simulink model "LQR"  (R2025b)
settings: Solver=VariableStepAuto  StartTime=0.0  StopTime=10  RelTol=1e-5
InitFcn:
  | clear; clc; close all;
  | 
  | % --- 1. System Parameters ---
  | m = 0.2;
  | M = 1;
  | g = 9.81;
  | bc = 0.1;
  | bp = 0.05;
  | l0 = 0.5;
  | theta0 = 0;
  | x0 = -0.5; % or -5
  | 
  | % --- 2. State-Space Matrices ---
  | A = [0, 1, 0, 0;
  |      0, -bc / M, (m * g) / M, bp / (M * l0);
  |      0, 0, 0, 1;
  |      0, bc / (M * l0), -g * (M + m) / (M * l0), -bp * (M + m) / (M * m * l0 ^ 2)];
  | 
  | % Only the 1st column of B is used (Input: Force F)
  | B_LQR = [0; 1 / M; 0; -1 / (M * l0)];
  | 
  | % --- 3. LQR Design ---
  | Q = diag([1000, 10, 500, 10]);
  | R = 1;
  | 
  | % Calculate LQR Gain 'K' silently
  | K = lqr(A, B_LQR, Q, R); % 31.6228   14.0488  -17.7264    0.3611
model workspace (MAT data in the model file):
  Sig = Simulink.Signal
  Sig.Dimensions = -1
  Sig.DimensionsMode = 'auto'
  Sig.Complexity = 'auto'
  Sig.SampleTime = -1
  Sig.SamplingMode = 'auto'
  Sig.DataType = 'auto'
undefined symbols (not defined in the file or in its folder): L, X, Y, Z
libraries: sm_lib x13, nesl_utility x7
settings Model: Creator=JNemune  LastModifiedBy=JNemune

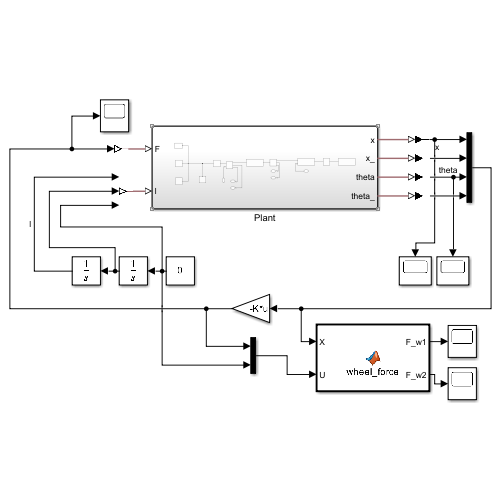
[thumbnail: Simulink's stored preview of the top-level diagram]
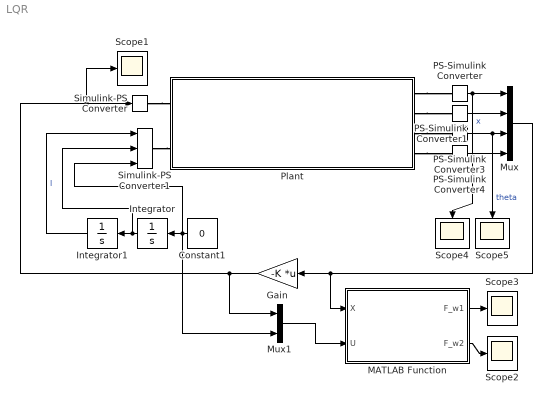
== system LQR ==
  Constant1 : Constant  Value=0
  Gain : Gain  Gain=-K  Multiplication=Matrix(K*u)
  Integrator : Integrator
  Integrator1 : Integrator  InitialCondition=l0
  MATLAB Function : MATLAB Function  TreatAsAtomicUnit=on
  Mux : Mux
  Mux1 : Mux  Inputs=2
  PS-Simulink Converter{,1,3..4} (4 alike) : nesl_utility/PS-Simulink Converter  PhysicalDomain=network_engine_domain  SubClassName=ps_output  LeftPortType=input  RightPortType=output  PseudoPeriodic=off  Frequencies=[]  VectorFormat=inherit  Unit=inherit  AffineConversion=off
  Plant : Subsystem
  Scope{1..5} (5 alike) : Scope
      Scope1 settings: Title=Plant Input (F, l_ddot)  ActiveDisplayYMinimum=-3.88186183734339  ActiveDisplayYMaximum=17.999527205084721
      Scope2 settings: Title=Plant Input (F, l_ddot)  ActiveDisplayYMinimum=5.7232322835325906  ActiveDisplayYMaximum=6.2250486767824951  DataLoggingVariableName=ScopeData2
      Scope3 settings: Title=Plant Input (F, l_ddot)  ActiveDisplayYMinimum=5.6634140711184715  ActiveDisplayYMaximum=6.09883492734478  DataLoggingVariableName=ScopeData3
      Scope4 settings: Title=Plant Input (F, l_ddot)  ActiveDisplayYMinimum=-0.56814105763095268  ActiveDisplayYMaximum=0.11326951867857375
      Scope5 settings: Title=Plant Input (F, l_ddot)  ActiveDisplayYMinimum=-0.29673612139259414  ActiveDisplayYMaximum=0.21369870792859819  DataLoggingVariableName=ScopeData4
  Simulink-PS Converter : nesl_utility/Simulink-PS Converter  PhysicalDomain=network_engine_domain  SubClassName=ps_input  LeftPortType=input  RightPortType=output  PseudoPeriodic=off  Frequencies=[]  NoiseDistribution=none  NoiseParameters=[]  Unit=1  AffineConversion=off  FilteringAndDerivatives=provide  SimscapeFilterOrder=1  InputFilterTimeConstant=0.001  UdotUserProvided=0
  Simulink-PS Converter1 : nesl_utility/Simulink-PS Converter  PhysicalDomain=network_engine_domain  SubClassName=ps_input  LeftPortType=input  RightPortType=output  PseudoPeriodic=off  Frequencies=[]  NoiseDistribution=none  NoiseParameters=[]  Unit=1  AffineConversion=off  FilteringAndDerivatives=provide  SimscapeFilterOrder=1  InputFilterTimeConstant=0.001  UdotUserProvided=2
  wires:
  Integrator/1 -> Simulink-PS Converter1/2, Integrator1/1
  Integrator1/1 -> Simulink-PS Converter1/1  "l"
  Constant1/1 -> Mux1/2, Simulink-PS Converter1/3, Integrator/1
  Gain/1 -> Mux1/1, Simulink-PS Converter/1, Scope1/1
  Mux/1 -> MATLAB Function/1(X), Gain/1
  PS-Simulink Converter1/1 -> Mux/2
  PS-Simulink Converter3/1 -> Scope5/1, Mux/3  "theta"
  PS-Simulink Converter4/1 -> Mux/4
  PS-Simulink Converter/1 -> Scope4/1, Mux/1  "x"
  Mux1/1 -> MATLAB Function/2(U)
  MATLAB Function/1(F_w1) -> Scope3/1
  MATLAB Function/2(F_w2) -> Scope2/1
  connections:
  Plant/RConn2 -- PS-Simulink Converter1/LConn1
  Simulink-PS Converter1/RConn1 -- Plant/LConn2
  Simulink-PS Converter/RConn1 -- Plant/LConn1
  Plant/RConn3 -- PS-Simulink Converter3/LConn1
  Plant/RConn1 -- PS-Simulink Converter/LConn1
  Plant/RConn4 -- PS-Simulink Converter4/LConn1

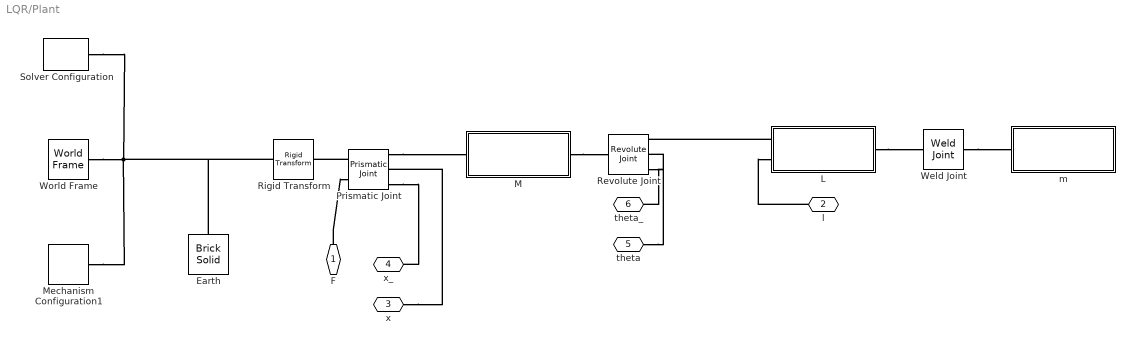
== system LQR/Plant ==
  Earth : sm_lib/Body Elements/Brick Solid  BrickDimensions=[1000 1 1]  BrickDimensionsUnits=mm  ExportEntireGeometry=off  InertiaType=CalculateFromGeometry  BasedOnType=Density  Density=1000  DensityUnits=kg/m^3  Mass=1  MassUnits=kg  CenterOfMass=[0 0 0]  CenterOfMassUnits=m  MomentsOfInertia=[1 1 1]  MomentsOfInertiaUnits=kg*m^2  ProductsOfInertia=[0 0 0]  ProductsOfInertiaUnits=kg*m^2  GraphicType=FromGeometry  MarkerShape=Sphere  MarkerSize=10  GraphicVisPropType=SimpleVisualProperties  GraphicDiffuseColor=[0.5 0.5 0.5]  GraphicOpacity=1.0  GraphicSpecularColor=[0.5 0.5 0.5 1.0]  GraphicAmbientColor=[0.15 0.15 0.15 1.0]  GraphicEmissiveColor=[0.0 0.0 0.0 1.0]  GraphicShininess=75  DoExposeReferenceFrame=on  SerializedFrames=<Frames/>
  L : Subsystem
  M : Subsystem
  Mechanism Configuration1 : sm_lib/Utilities/Mechanism Configuration  UniformGravity=Constant  GravityVector=[0 0 -g]  GravityVectorUnits=m/s^2  LinearizationDelta=0.001  JointModeTransitionNonlinearIterations=2
  Prismatic Joint : sm_lib/Joints/Prismatic Joint  JointMode=Normal  CompositeWrenchDir=FollowerOnBase  CompositeWrenchFrame=BaseFrame  SenseConstraintForce=off  SenseConstraintTorque=off  SenseTotalForce=off  SenseTotalTorque=off  PositionTargetSpecify=on  PositionTargetPriority=High  PositionTargetValue=x0  PositionTargetValueUnits=m  VelocityTargetSpecify=off  VelocityTargetPriority=High  VelocityTargetValue=0  VelocityTargetValueUnits=m/s  EquilibriumPosition=0  EquilibriumPositionUnits=m  SpringStiffness=0  SpringStiffnessUnits=N/m  DampingCoefficient=bc  DampingCoefficientUnits=N/(m/s)  LowerLimitSpecify=off  LowerLimitBound=-1  LowerLimitBoundUnits=m  LowerLimitStiffness=1e6  LowerLimitStiffnessUnits=N/m  LowerLimitDamping=1e3  LowerLimitDampingUnits=N/(m/s)  LowerLimitTransitionRegionWidth=1e-4  LowerLimitTransitionRegionWidthUnits=m  UpperLimitSpecify=off  UpperLimitBound=1  UpperLimitBoundUnits=m  UpperLimitStiffness=1e6  UpperLimitStiffnessUnits=N/m  UpperLimitDamping=1e3  UpperLimitDampingUnits=N/(m/s)  UpperLimitTransitionRegionWidth=1e-4  UpperLimitTransitionRegionWidthUnits=m  TorqueActuationMode=InputTorque  MotionActuationMode=ComputedMotion  SensePosition=on  SenseVelocity=on  SenseAcceleration=off  SenseTorqueForce=off  SenseLowerLimitTorqueForce=off  SenseUpperLimitTorqueForce=off
  Revolute Joint : sm_lib/Joints/Revolute Joint  JointMode=Normal  CompositeWrenchDir=FollowerOnBase  CompositeWrenchFrame=BaseFrame  SenseConstraintForce=off  SenseConstraintTorque=off  SenseTotalForce=off  SenseTotalTorque=off  PositionTargetSpecify=on  PositionTargetPriority=High  PositionTargetValue=theta0  PositionTargetValueUnits=rad  VelocityTargetSpecify=off  VelocityTargetPriority=High  VelocityTargetValue=0  VelocityTargetValueUnits=deg/s  EquilibriumPosition=0  EquilibriumPositionUnits=deg  SpringStiffness=0  SpringStiffnessUnits=N*m/deg  DampingCoefficient=bp  DampingCoefficientUnits=N*m*s/rad  LowerLimitSpecify=off  LowerLimitBound=-90  LowerLimitBoundUnits=deg  LowerLimitStiffness=1e4  LowerLimitStiffnessUnits=N*m/deg  LowerLimitDamping=10  LowerLimitDampingUnits=N*m/(deg/s)  LowerLimitTransitionRegionWidth=0.1  LowerLimitTransitionRegionWidthUnits=deg  UpperLimitSpecify=off  UpperLimitBound=90  UpperLimitBoundUnits=deg  UpperLimitStiffness=1e4  UpperLimitStiffnessUnits=N*m/deg  UpperLimitDamping=10  UpperLimitDampingUnits=N*m/(deg/s)  UpperLimitTransitionRegionWidth=0.1  UpperLimitTransitionRegionWidthUnits=deg  TorqueActuationMode=NoTorque  MotionActuationMode=ComputedMotion  SensePosition=on  SenseVelocity=on  SenseAcceleration=off  SenseTorqueForce=off  SenseLowerLimitTorqueForce=off  SenseUpperLimitTorqueForce=off
  Rigid Transform : sm_lib/Frames and Transforms/Rigid Transform  RotationMethod=StandardAxis  FollAlignAxisA=+X  BaseAlignAxisA=+Y  FollAlignAxisB=+Y  BaseAlignAxisB=+Z  RotationStandardAxis=+Y  RotationAngle=90  RotationAngleUnits=deg  RotationArbitraryAxis=[0 0 1]  RotationSequenceAxes=FollowerAxes  RotationSequence=XYX  RotationSequenceAngles=[0 0 0]  RotationSequenceAnglesUnits=deg  RotationMatrix=[1 0 0; 0 1 0; 0 0 1]  Quaternion=[1 0 0 0]  TranslationMethod=None  TranslationCartesianOffset=[x0 0 0]  TranslationCartesianOffsetUnits=m  TranslationStandardAxis=+Z  TranslationStandardOffset=0  TranslationStandardOffsetUnits=m  TranslationROffset=0  TranslationROffsetUnits=m  TranslationThetaOffset=0  TranslationThetaOffsetUnits=deg  TranslationZOffset=0  TranslationZOffsetUnits=m
  Solver Configuration : nesl_utility/Solver Configuration  PhysicalDomain=network_engine_domain  SubClassName=solver  LeftPortType=input  RightPortType=generic  Tones=[]  Harmonics=[]  SimulateNoise=off  Profile=off  UseLocalSampling=off  EnableSwitchedLinearOptims=on  FrequencyDomain=off  UseCCode=off  RelTol=0.001  AbsTol=0.001  MinStep=1e-09  ToWorkspace=off  RevertToSquareIcSolve=off  NumHomotopyIterations=100  PhasorMode=off  PhasorModeNumHarmonics=1  ConsistencySolver=NEWTON_XTOL_AFTER_FTOL  IndexReductionMethod=DerivativeReplacement  DoDC=off  ResidualTolerance=1e-09  ConsistencyTolSource=GLOBAL  ConsistencyAbsTol=0.001  ConsistencyRelTol=0.001  ConsistencyTolFactor=0.001  UseLocalSolver=off  LocalSolverChoice=NE_BACKWARD_EULER_ADVANCER  ResolveIndetEquations=on  FunctionEvalNumThread=1  LocalSolverSampleTime=0.001  DoFixedCost=off  MaxNonlinIter=3  MaxModeIter=2  ComputeImpulses=off  ImpulseIterations=2  LinearAlgebra=auto  LinearAlgebraNumThread=0  EquationFormulation=NE_TIME_EF  DelaysMemoryBudget=1024  AutomaticFiltering=on  FilteringTimeConstant=0.001  PartitionStorageMethod=AS_NEEDED  PartitionMemoryBudget=1024  PartitionMethod=ROBUST  MultibodyUseLocalSolver=off  MultibodyLocalSolverChoice=ODE1  MultibodyLocalSolverSampleTime=0.001
  Weld Joint : sm_lib/Joints/Weld Joint  JointMode=Normal  CompositeWrenchDir=FollowerOnBase  CompositeWrenchFrame=BaseFrame  SenseConstraintForce=off  SenseConstraintTorque=off  SenseTotalForce=off  SenseTotalTorque=off
  World Frame : sm_lib/Frames and Transforms/World Frame
  m : Subsystem
  F : PMIOPort  Side=Left
  l : PMIOPort  Port=2  Side=Left
  x : PMIOPort  Port=3  Side=Right
  x_ : PMIOPort  Port=4  Side=Right
  theta : PMIOPort  Port=5  Side=Right
  theta_ : PMIOPort  Port=6  Side=Right
  connections:
  Solver Configuration/RConn1 -- Earth/RConn1 -- Rigid Transform/LConn1 -- World Frame/RConn1 -- Mechanism Configuration1/RConn1
  Prismatic Joint/LConn1 -- Rigid Transform/RConn1
  Weld Joint/RConn1 -- m/LConn1
  L/LConn1 -- Revolute Joint/RConn1
  M/RConn1 -- Revolute Joint/LConn1
  L/RConn1 -- Weld Joint/LConn1
  Prismatic Joint/RConn1 -- M/LConn1
  l/RConn1 -- L/LConn2
  F/RConn1 -- Prismatic Joint/LConn2
  Revolute Joint/RConn3 -- theta_/RConn1
  Prismatic Joint/RConn3 -- x_/RConn1
  x/RConn1 -- Prismatic Joint/RConn2
  theta/RConn1 -- Revolute Joint/RConn2

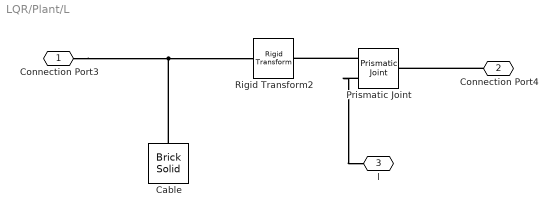
== system LQR/Plant/L ==
  Cable : sm_lib/Body Elements/Brick Solid  BrickDimensions=[l0, 0.001, 0.001]  BrickDimensionsUnits=m  ExportEntireGeometry=off  InertiaType=Custom  BasedOnType=Density  Density=1000  DensityUnits=kg/m^3  Mass=0  MassUnits=kg  CenterOfMass=[0 0 0]  CenterOfMassUnits=m  MomentsOfInertia=[0 0 0]  MomentsOfInertiaUnits=kg*m^2  ProductsOfInertia=[0 0 0]  ProductsOfInertiaUnits=kg*m^2  GraphicType=FromGeometry  MarkerShape=Frame  MarkerSize=10  GraphicVisPropType=SimpleVisualProperties  GraphicDiffuseColor=[0.5 0.5 0.5]  GraphicOpacity=1.0  GraphicSpecularColor=[0.5 0.5 0.5 1.0]  GraphicAmbientColor=[0.15 0.15 0.15 1.0]  GraphicEmissiveColor=[0.0 0.0 0.0 1.0]  GraphicShininess=75  DoExposeReferenceFrame=off  SerializedFrames=|
      | <Frames>
      | 
      |   <Frame>
      |     <Id>Frame1</Id>
      |     <Value>
      |       <Name>cable joint</Name>
      |       <Origin>
      |         <Source>GeometricFeature</Source>
      |         <FeatureName>-x -y +z point</FeatureName>
      |       </Origin>
      |       <PrimaryAxis>
      |         <DefinedDirection>+Z</DefinedDirection>
      |         <Source>ReferenceFrame</Source>
      |         <SourceDirection>+Z</SourceDirection>
      |         <FeatureName></FeatureName>
      |       </PrimaryAxis>
      |       <SecondaryAxis>
      |         <DefinedDirection>+X</DefinedDirection>
      |         <Source>ReferenceFrame</Source>
      |         <SourceDirection>+X</SourceDirection>
      |         <FeatureName></FeatureName>
      |       </SecondaryAxis>
      |     </Value>
      |   </Frame>
      | 
      | </Frames>
  Prismatic Joint : sm_lib/Joints/Prismatic Joint  JointMode=Normal  CompositeWrenchDir=FollowerOnBase  CompositeWrenchFrame=BaseFrame  SenseConstraintForce=off  SenseConstraintTorque=off  SenseTotalForce=off  SenseTotalTorque=off  PositionTargetSpecify=off  PositionTargetPriority=High  PositionTargetValue=l0  PositionTargetValueUnits=m  VelocityTargetSpecify=off  VelocityTargetPriority=High  VelocityTargetValue=0  VelocityTargetValueUnits=m/s  EquilibriumPosition=0  EquilibriumPositionUnits=m  SpringStiffness=0  SpringStiffnessUnits=N/m  DampingCoefficient=0  DampingCoefficientUnits=N/(m/s)  LowerLimitSpecify=off  LowerLimitBound=-1  LowerLimitBoundUnits=m  LowerLimitStiffness=1e6  LowerLimitStiffnessUnits=N/m  LowerLimitDamping=1e3  LowerLimitDampingUnits=N/(m/s)  LowerLimitTransitionRegionWidth=1e-4  LowerLimitTransitionRegionWidthUnits=m  UpperLimitSpecify=off  UpperLimitBound=1  UpperLimitBoundUnits=m  UpperLimitStiffness=1e6  UpperLimitStiffnessUnits=N/m  UpperLimitDamping=1e3  UpperLimitDampingUnits=N/(m/s)  UpperLimitTransitionRegionWidth=1e-4  UpperLimitTransitionRegionWidthUnits=m  TorqueActuationMode=ComputedTorque  MotionActuationMode=InputMotion  SensePosition=off  SenseVelocity=off  SenseAcceleration=off  SenseTorqueForce=off  SenseLowerLimitTorqueForce=off  SenseUpperLimitTorqueForce=off
  Rigid Transform2 : sm_lib/Frames and Transforms/Rigid Transform  RotationMethod=StandardAxis  FollAlignAxisA=+X  BaseAlignAxisA=+Y  FollAlignAxisB=+Y  BaseAlignAxisB=+Z  RotationStandardAxis=+Y  RotationAngle=pi/2  RotationAngleUnits=rad  RotationArbitraryAxis=[0 0 1]  RotationSequenceAxes=FollowerAxes  RotationSequence=XYX  RotationSequenceAngles=[0 0 0]  RotationSequenceAnglesUnits=deg  RotationMatrix=[1 0 0; 0 1 0; 0 0 1]  Quaternion=[1 0 0 0]  TranslationMethod=None  TranslationCartesianOffset=[L/2*cos(theta0), L/2*sin(theta0), 0]  TranslationCartesianOffsetUnits=m  TranslationStandardAxis=+Z  TranslationStandardOffset=0  TranslationStandardOffsetUnits=m  TranslationROffset=0  TranslationROffsetUnits=m  TranslationThetaOffset=0  TranslationThetaOffsetUnits=deg  TranslationZOffset=0  TranslationZOffsetUnits=m
  Connection Port3 : PMIOPort  Side=Left
  Connection Port4 : PMIOPort  Port=2  Side=Right
  l : PMIOPort  Port=3  Side=Left
  connections:
  Prismatic Joint/LConn1 -- Rigid Transform2/RConn1
  Connection Port3/RConn1 -- Cable/LConn1 -- Rigid Transform2/LConn1
  Connection Port4/RConn1 -- Prismatic Joint/RConn1
  Prismatic Joint/LConn2 -- l/RConn1

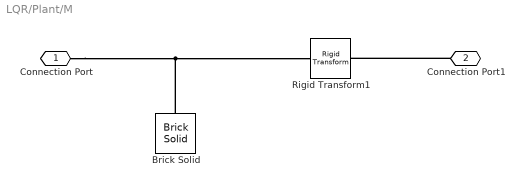
== system LQR/Plant/M ==
  Brick Solid : sm_lib/Body Elements/Brick Solid  BrickDimensions=[1 1 1]  BrickDimensionsUnits=mm  ExportEntireGeometry=off  InertiaType=PointMass  BasedOnType=Density  Density=1000  DensityUnits=kg/m^3  Mass=M  MassUnits=kg  CenterOfMass=[0 0 0]  CenterOfMassUnits=m  MomentsOfInertia=[1 1 1]  MomentsOfInertiaUnits=kg*m^2  ProductsOfInertia=[0 0 0]  ProductsOfInertiaUnits=kg*m^2  GraphicType=FromGeometry  MarkerShape=Sphere  MarkerSize=10  GraphicVisPropType=SimpleVisualProperties  GraphicDiffuseColor=[0.5 0.5 0.5]  GraphicOpacity=1.0  GraphicSpecularColor=[0.5 0.5 0.5 1.0]  GraphicAmbientColor=[0.15 0.15 0.15 1.0]  GraphicEmissiveColor=[0.0 0.0 0.0 1.0]  GraphicShininess=75  DoExposeReferenceFrame=on  SerializedFrames=<Frames/>
  Rigid Transform1 : sm_lib/Frames and Transforms/Rigid Transform  RotationMethod=StandardAxis  FollAlignAxisA=+X  BaseAlignAxisA=+Y  FollAlignAxisB=+Y  BaseAlignAxisB=+Z  RotationStandardAxis=+X  RotationAngle=90  RotationAngleUnits=deg  RotationArbitraryAxis=[0 0 1]  RotationSequenceAxes=FollowerAxes  RotationSequence=XYX  RotationSequenceAngles=[0 0 0]  RotationSequenceAnglesUnits=deg  RotationMatrix=[1 0 0; 0 1 0; 0 0 1]  Quaternion=[1 0 0 0]  TranslationMethod=None  TranslationCartesianOffset=[0 0 0]  TranslationCartesianOffsetUnits=m  TranslationStandardAxis=+Z  TranslationStandardOffset=0  TranslationStandardOffsetUnits=m  TranslationROffset=0  TranslationROffsetUnits=m  TranslationThetaOffset=0  TranslationThetaOffsetUnits=deg  TranslationZOffset=0  TranslationZOffsetUnits=m
  Connection Port : PMIOPort  Side=Left
  Connection Port1 : PMIOPort  Port=2  Side=Right
  connections:
  Brick Solid/RConn1 -- Connection Port/RConn1 -- Rigid Transform1/LConn1
  Connection Port1/RConn1 -- Rigid Transform1/RConn1

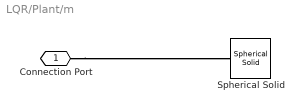
== system LQR/Plant/m ==
  Spherical Solid : sm_lib/Body Elements/Spherical Solid  SphereRadius=1  SphereRadiusUnits=cm  ExportEntireGeometry=off  InertiaType=PointMass  BasedOnType=Density  Density=1000  DensityUnits=kg/m^3  Mass=m  MassUnits=kg  CenterOfMass=[0 0 0]  CenterOfMassUnits=m  MomentsOfInertia=[1 1 1]  MomentsOfInertiaUnits=kg*m^2  ProductsOfInertia=[0 0 0]  ProductsOfInertiaUnits=kg*m^2  GraphicType=FromGeometry  MarkerShape=Sphere  MarkerSize=10  GraphicVisPropType=SimpleVisualProperties  GraphicDiffuseColor=[0.5 0.5 0.5]  GraphicOpacity=1.0  GraphicSpecularColor=[0.5 0.5 0.5 1.0]  GraphicAmbientColor=[0.15 0.15 0.15 1.0]  GraphicEmissiveColor=[0.0 0.0 0.0 1.0]  GraphicShininess=75  DoExposeReferenceFrame=on  SerializedFrames=<Frames/>
  Connection Port : PMIOPort  Side=Left
  connections:
  Connection Port/RConn1 -- Spherical Solid/RConn1

== matlab function LQR/MATLAB Function ==
  data: X input; F_w1 output; U input; F_w2 output
function [F_w1, F_w2] = wheel_force(X, U)
    % Extract mechanical states for LQR architecture
    x_dot = X(2);
    theta = X(3);
    theta_dot = X(4);

    % Define constant cable parameters
    l = 0.5;
    l_dot = 0;

    % Extract inputs
    F = U(1);
    l_ddot = U(2);

    % System physical parameters
    m = 0.2;
    M = 1.0;
    g = 9.81;
    bc = 0.1;
    bp = 0.05;
    D1 = 0.2;
    D2 = 0.1;

    % Precompute trigonometric terms
    s = sin(theta);
    c = cos(theta);

    % Calculate theta_ddot using analytical inversion
    RHS1 = F - bc * x_dot - m * l_ddot * s ...
        - 2 * m * l_dot * theta_dot * c ...
        + m * l * theta_dot ^ 2 * s;

    RHS2 = -2 * m * l * l_dot * theta_dot ...
        - m * g * l * s ...
        - bp * theta_dot;

    theta_ddot = ((M + m) * RHS2 - m * l * c * RHS1) / (m * l ^ 2 * (M + m * s ^ 2));

    % Payload vertical acceleration via local polar coordinates
    a_radial = l_ddot - l * theta_dot ^ 2;
    a_tang = l * theta_ddot + 2 * l_dot * theta_dot;
    y_p_ddot = -a_radial * c + a_tang * s;

    % Wheel load calculations
    F_sum = (M + m) * g + m * y_p_ddot;
    F_diff = (D2 * bc * x_dot - bp * theta_dot) / D1;

    % Final vertical loads on left and right wheel sets
    F_w1 = (F_sum - F_diff) / 2;
    F_w2 = (F_sum + F_diff) / 2;
end
